simulink model "car_model"  (R2025a)
settings: Solver=ode3  StartTime=0.0  StopTime=inf  FixedStep=0.01  RelTol=1e-3  EnableMultiTasking=on
model workspace (MAT data in the model file):
  A = Simulink.Parameter
  A.Value = 2.4
  A.Complexity = 'real'
  A.Dimensions = [1 1]
  A.DataType = 'auto'
  Cd = Simulink.Parameter
  Cd.Value = 0.32
  Cd.Complexity = 'real'
  Cd.Dimensions = [1 1]
  Cd.DataType = 'auto'
  Cr = Simulink.Parameter
  Cr.Value = 0.01
  Cr.Complexity = 'real'
  Cr.Dimensions = [1 1]
  Cr.DataType = 'auto'
  Tm = Simulink.Parameter
  Tm.Value = 190
  Tm.Complexity = 'real'
  Tm.Dimensions = [1 1]
  Tm.DataType = 'auto'
  betac = Simulink.Parameter
  betac.Value = 0.4
  betac.Complexity = 'real'
  betac.Dimensions = [1 1]
  betac.DataType = 'auto'
  g = Simulink.Parameter
  g.Value = 9.8
  g.Complexity = 'real'
  g.Dimensions = [1 1]
  g.DataType = 'auto'
  m = Simulink.Parameter
  m.Value = 1000
  m.Complexity = 'real'
  m.Dimensions = [1 1]
  m.DataType = 'auto'
  omegam = Simulink.Parameter
  omegam.Value = 420
  omegam.Complexity = 'real'
  omegam.Dimensions = [1 1]
  omegam.DataType = 'auto'
  rho = Simulink.Parameter
  rho.Value = 1.2
  rho.Complexity = 'real'
  rho.Dimensions = [1 1]
  rho.DataType = 'auto'
libraries: simulink x2, simulink_extras x1
settings Model: Creator=root  LastModifiedBy=Taka
settings SolverCC: ShapePreserveControl=EnableAll  AlgebraicLoopSolver=TrustRegion
settings OptimizationCC: DefaultUnderspecifiedDataType=single  EfficientFloat2IntCast=on  LifeSpan=inf
settings DebuggingCC: UnconnectedInputMsg=warning  UnconnectedOutputMsg=warning  UnconnectedLineMsg=warning  SFUnexpectedBacktrackingDiag=warning  SFNoUnconditionalDefaultTransitionDiag=warning  SFExecutionAtInitializationDiag=none  ArithmeticOperatorsInVariantConditions=warning
settings HardwareCC: ProdBitPerSizeT=32.0  ProdBitPerPtrDiffT=32.0  ProdWordSize=32.0  ProdHWDeviceType=Specified
settings ModelReferenceCC: EnableRefExpFcnMdlSchedulingChecks=on  PropagateSignalLabelsOutOfModel=off
settings SFSimCC: SimUseLocalCustomCode=off  CustomCodeUndefinedFunction=UseInterfaceOnly
settings RTWCC: RTWUseLocalCustomCode=off  GPUComputeCapability=3.5
settings CodeAppCC: StateflowObjectComments=on
settings GRTTargetCC: TargetLangStandard=C89/C90 (ANSI)
settings ConfigComp: CovMetricSettings=dw  CovSaveCumulativeToWorkspaceVar=on  CovSaveSingleToWorkspaceVar=on  CovExternalEMLEnable=off
settings CustomCC: propDiagFcnCallOutput=2  propDiagAttribOutput=2  propIdentEvents=0  SimEventsActiveTab=0  propDiagStatOutput=2  propDiagChangeAttrib=2  propIdentEventSeed=123456789  propPreventDuplicateEvents=1  propRNGIdenticalSeeds=1  propMaxDesMdlSimulEvents=100000  propMaxDesBlkSimulEvents=1000
settings SimscapeCC: SimscapeNormalizeSystem=off
settings ConfigurationSet: Description=SimMechanics 2G

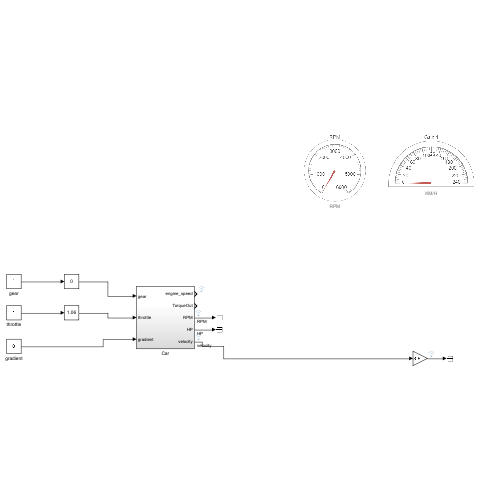
[thumbnail: Simulink's stored preview of the top-level diagram]
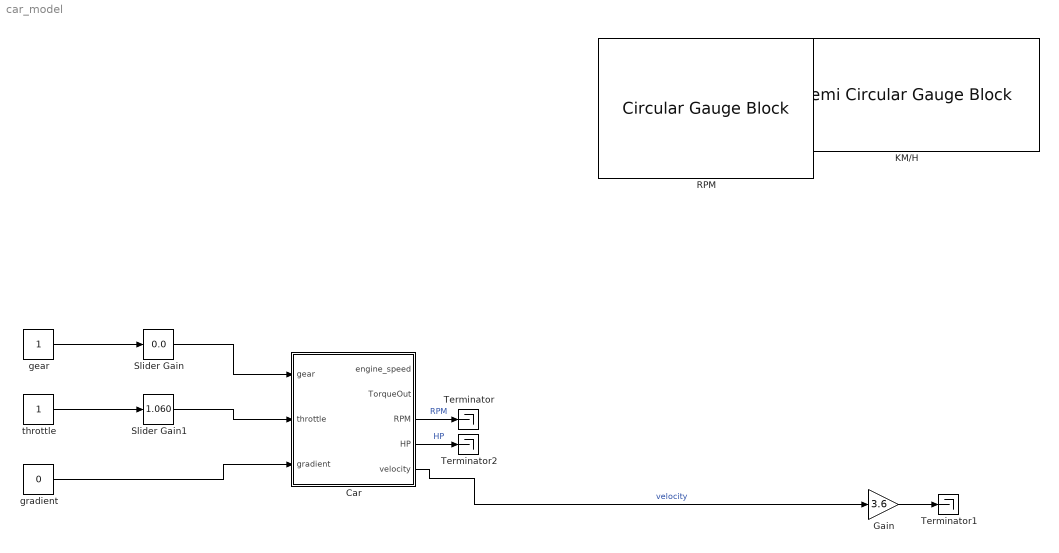
== system car_model ==
  Car : Subsystem
  Gain : Gain  Gain=3.6
  KM/H : SemiCircularGaugeBlock  ScaleMax=240  TickInterval=20  FontColor=[0.0, 0.0, 0.0]
  RPM : CircularGaugeBlock  ScaleMax=6000  FontColor=[0.0, 0.0, 0.0]
  Slider Gain : simulink/Math Operations/Slider Gain  gain=0.0  low=0  high=5
  Slider Gain1 : simulink/Math Operations/Slider Gain  gain=1.060  low=-0.05  high=1.06
  Terminator : Terminator
  Terminator1 : Terminator
  Terminator2 : Terminator
  gear : Constant
  gradient : Constant  Value=0
  throttle : Constant
  wires:
  Car/5(velocity) -> Gain/1  "velocity"
  Car/3(RPM) -> Terminator/1  "RPM"
  Gain/1 -> Terminator1/1
  Car/4(HP) -> Terminator2/1  "HP"
  gradient/1 -> Car/3(gradient)
  gear/1 -> Slider Gain/1
  Slider Gain/1 -> Car/1(gear)
  throttle/1 -> Slider Gain1/1
  Slider Gain1/1 -> Car/2(throttle)

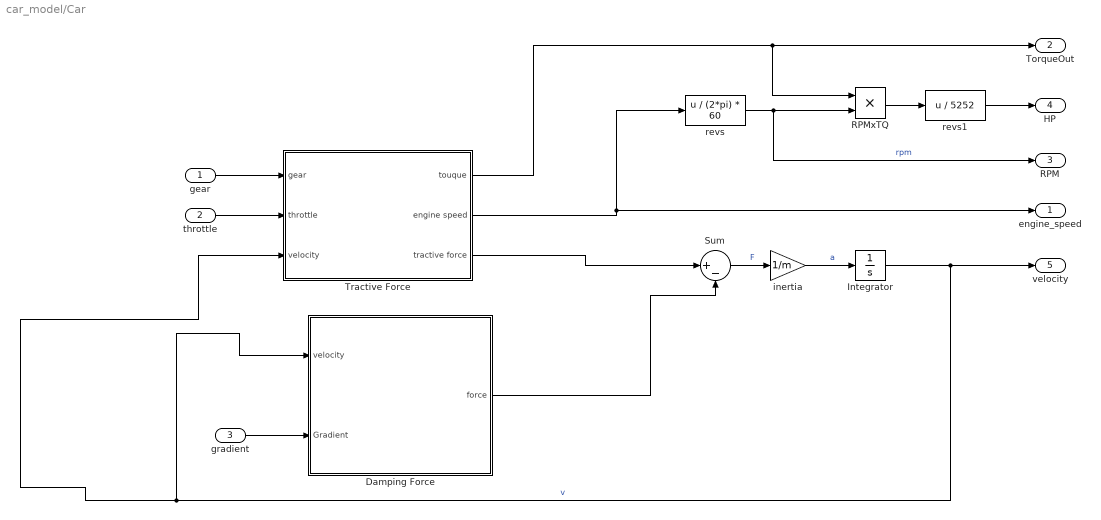
== system car_model/Car ==
  gear : Inport
  throttle : Inport  Port=2  OutMin=0  OutMax=1
  gradient : Inport  Port=3
  Damping Force : Subsystem
  Integrator : Integrator
  RPMxTQ : Product
  Sum : Sum  Inputs=|+-
  Tractive Force : Subsystem
  inertia : Gain  Gain=1/m
  revs : Fcn  Expr=u / (2*pi) * 60
  revs1 : Fcn  Expr=u / 5252
  engine_speed : Outport  VectorParamsAs1DForOutWhenUnconnected=off
  TorqueOut : Outport  Port=2  VectorParamsAs1DForOutWhenUnconnected=off
  RPM : Outport  Port=3  VectorParamsAs1DForOutWhenUnconnected=off
  HP : Outport  Port=4  VectorParamsAs1DForOutWhenUnconnected=off
  velocity : Outport  Port=5  VectorParamsAs1DForOutWhenUnconnected=off
  wires:
  inertia/1 -> Integrator/1  "a"
  Sum/1 -> inertia/1  "F"
  Integrator/1 -> Tractive Force/3(velocity), Damping Force/1(velocity), velocity/1  "v"
  revs/1 -> RPM/1, RPMxTQ/2  "rpm"
  RPMxTQ/1 -> revs1/1
  revs1/1 -> HP/1
  Tractive Force/2(engine speed) -> revs/1, engine_speed/1
  Tractive Force/1(touque) -> TorqueOut/1, RPMxTQ/1
  gear/1 -> Tractive Force/1(gear)
  throttle/1 -> Tractive Force/2(throttle)
  Tractive Force/3(tractive force) -> Sum/1
  gradient/1 -> Damping Force/2(Gradient)
  Damping Force/1(force) -> Sum/2

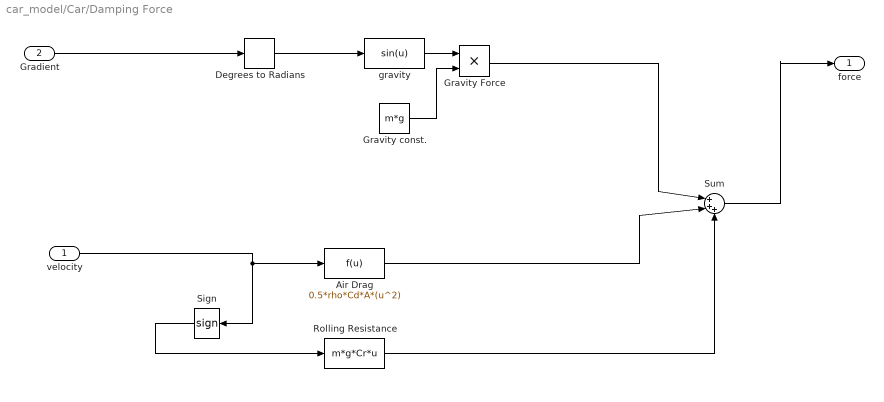
== system car_model/Car/Damping Force ==
  velocity : Inport
  Gradient : Inport  Port=2
  Air Drag : Fcn  Expr=0.5*rho*Cd*A*(u^2)
  Degrees to Radians : simulink_extras/Transformations/Degrees to Radians
  Gravity Force : Product
  Gravity const. : Constant  Value=m*g
  Rolling Resistance : Fcn  Expr=m*g*Cr*u
  Sign : Signum
  Sum : Sum  Inputs=|+++
  gravity : Fcn  Expr=sin(u)
  force : Outport  VectorParamsAs1DForOutWhenUnconnected=off
  wires:
  Sign/1 -> Rolling Resistance/1
  Rolling Resistance/1 -> Sum/3
  Gravity const./1 -> Gravity Force/2
  Gradient/1 -> Degrees to Radians/1
  Degrees to Radians/1 -> gravity/1
  gravity/1 -> Gravity Force/1
  Air Drag/1 -> Sum/2
  Gravity Force/1 -> Sum/1
  velocity/1 -> Air Drag/1, Sign/1
  Sum/1 -> force/1

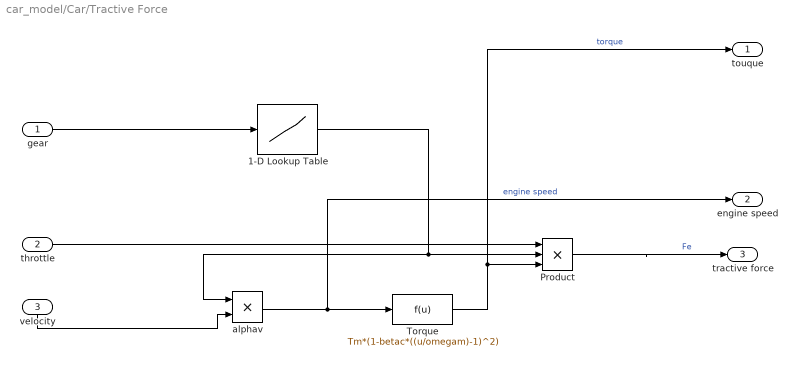
== system car_model/Car/Tractive Force ==
  gear : Inport
  throttle : Inport  Port=2
  velocity : Inport  Port=3
  1-D Lookup Table : Lookup_n-D  NumberOfTableDimensions=1  BreakpointsForDimension1=int16([1,2,3,4,5]);  Table=int16([40,25,16,12,10]);  InternalRulePriority=Speed  RndMeth=Simplest
  Product : Product  Inputs=3
  Torque : Fcn  Expr=Tm*(1-betac*((u/omegam)-1)^2)
  alphav : Product
  touque : Outport  VectorParamsAs1DForOutWhenUnconnected=off
  engine speed : Outport  Port=2  VectorParamsAs1DForOutWhenUnconnected=off
  tractive force : Outport  Port=3  VectorParamsAs1DForOutWhenUnconnected=off
  wires:
  gear/1 -> 1-D Lookup Table/1
  Torque/1 -> touque/1, Product/3  "torque"
  throttle/1 -> Product/1
  1-D Lookup Table/1 -> Product/2, alphav/1
  alphav/1 -> engine speed/1, Torque/1  "engine speed"
  Product/1 -> tractive force/1  "Fe"
  velocity/1 -> alphav/2
